simulink model "testSetTorques2"  (Simulink 7.9)
settings: Solver=ode3  StartTime=0.0  StopTime=inf  FixedStep=1  RelTol=1e-3
undefined symbols (not defined in the file or in its folder): hFixed
libraries: utility x1
settings Model: Creator=jorhabib  LastModifiedBy=jorhabib

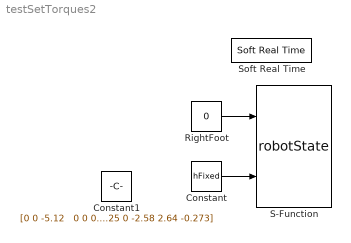
== system testSetTorques2 ==
  Constant : Constant  Value=hFixed  SampleTime=-1
  Constant1 : Constant  Value="[0 0 -5.12   0 0 0 0 0   -1.826 1.415 -0.216 0.810 0.018 -2.659 -0.49 0 -2.73 2.8 -0.273 -2.51 -0.25 0 -2.58 2.64 -0.273]"  SampleTime=-1
  RightFoot : Constant  Value=0  OutDataTypeStr=int8  SampleTime=-1
  S-Function : S-Function  FunctionName=robotState  Parameters=6,'icubGazeboSim','simulink'  EnableBusSupport=off
  Soft Real Time : utility/Soft Real Time  x=0.01
  wires:
  RightFoot/1 -> S-Function/1
  Constant/1 -> S-Function/2
